simulink model "BugE_v0_40_MAS_loads_reg"  (R2015b)
settings: Solver=FixedStepDiscrete  StartTime=0.0  StopTime=1370  FixedStep=sample_time  RelTol=1e-3
values from neighbouring files (symbols this model uses):
  AB_diode_dV = 0.9    [main_sync.m]
  air_density = 1.225    [main_sync.m]
  bus_ac_Pmax_abs = 240    [main_sync.m]
  bus_charger_Pmax = 1000    [main_sync.m]
  bus_load_Pmax_abs = 260    [main_sync.m]
  capInitVolt = capVmax*sqrt(capInitSoC)    [main_sync.m]
  cyc_kph = [cyc_kph(:,1), cyc_kph(:,2)*speed_max_limit/speed_max]    [main_sync.m]
  cyc_repeat = 0    [main_sync.m]
  ess1_init_soc = 1    [main_sync.m]
  ess1_soh = 1    [main_sync.m]
  ess2_init_soc = 1    [main_sync.m]
  ess2_soh = 1    [main_sync.m]
  ess3_init_soc = 1    [main_sync.m]
  ess3_soh = 1    [main_sync.m]
  ess4_init_soc = 1    [main_sync.m]
  ess4_soh = 1    [main_sync.m]
  ess5_init_soc = 1    [main_sync.m]
  ess5_soh = 1    [main_sync.m]
  gear_ratio = 6    [main_sync.m]
  JADE_on = 0    [main_sync.m]
  loadpower = rawcsv(:,2)    [main_sync.m]
  loadtime = rawcsv(:,1)    [main_sync.m]
  lockSOCs = 0    [main_sync.m]
  max_brk_torque = 300    [main_sync.m]
  no_wheels = 3    [main_sync.m]
  period2 = max(loadtime)    [main_sync.m]
  PV_Pmax = 100    [main_sync.m]
  sample_time = 0.01    [main_sync.m]
  startup_seq_step_delay = 0.2    [main_sync.m]
  stop_option = 0    [main_sync.m]
  use_drive_cycle = 1    [main_sync.m]
  use_real_subs_loads = 1    [main_sync.m]
  vbus_max = 25    [main_sync.m]
  vbus_min = 17    [main_sync.m]
  vbus_safety_threshold = 2    [main_sync.m]
  vbus_threshold = 20    [main_sync.m]
  veh_CD = 0.35    [main_sync.m]
  veh_FA = 1.543    [main_sync.m]
  veh_gravity = 9.81*veh_mass    (= 1863.9)    [main_sync.m]
  veh_mass = 190    [main_sync.m]
  wh_1st_rrc = 0.02    [main_sync.m]
  wh_bearing_frc = 0.0015    [main_sync.m]
  wh_inertia = 0.0556    [main_sync.m]
  wh_radius = 0.508/2    (= 0.254)    [main_sync.m]
undefined symbols (not defined in the file or in its folder): capC, capR, cyc_acc, cyc_avg_time_samples, cyc_brk, cyc_grade, cyc_key, DCM_eff_factor_for_Vin, DCM_eff_for_Iout, DCM_Iout, DCM_Iout_max, DCM_Pin_noload, DCM_Pout_max, DCM_Vin, DCM_Vout, DiscIntNeverNeededParam, ess2_coulombic_eff, ess2_Ineg_max_SOC, ess2_Ineg_max_temp, ess2_Ipos_max_SOC, ess2_Ipos_max_temp, ess2_max_ah_cap, ess2_max_volts, ess2_min_volts, ess2_module_parallel, ess2_module_series, ess2_r_dis, ess2_soc, ess2_SOC_for_Ilimit, ess2_temp_for_Ilimit, ess2_temp_max, ess2_tmp, ess2_voc, ess3_coulombic_eff, ess3_max_ah_cap, ess3_module_parallel, ess3_module_series, ess3_r_dis, ess3_soc, ess3_tmp, ess3_voc, ess_coulombic_eff, ess_Ineg_max_SOC, ess_Ineg_max_temp, ess_Ipos_max_SOC, ess_Ipos_max_temp, ess_max_ah_cap, ess_max_volts, ess_min_volts, ess_module_parallel, ess_module_series, ess_nominal_volts, ess_r_dis, ess_soc, ess_SOC_for_Ilimit, ess_temp_for_Ilimit, ess_temp_max, ess_tmp, ess_voc, MC_eff1 ... (+18)
libraries: simulink x140, commfilt2 x1, simulink_extras x1
(part 3 of 7)

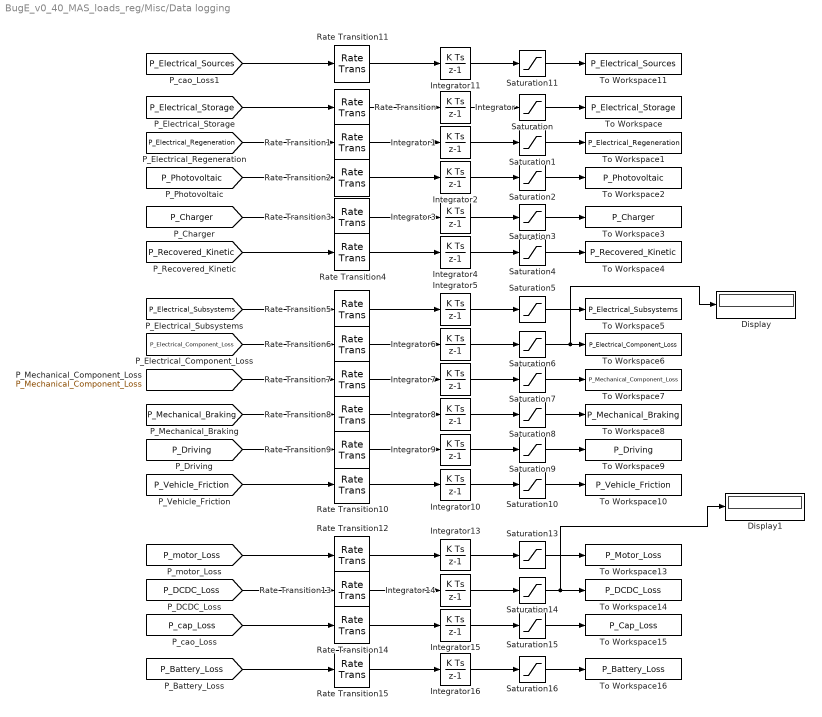
== system BugE_v0_40_MAS_loads_reg/Misc/Data logging ==
  Display : Display
  Display1 : Display
  Integrator{,1..11,13..16} (16 alike) : DiscreteIntegrator  InitialConditionSetting=State (most efficient)  ICPrevOutput=DiscIntNeverNeededParam  ICPrevScaledInput=DiscIntNeverNeededParam
  Rate Transition{,1..15} (16 alike) : RateTransition
  Saturation{,1..11,13..16} (16 alike) : Saturate  UpperLimit=inf  LowerLimit=0
  To Workspace : ToWorkspace  VariableName=P_Electrical_Storage  SampleTime=-1
      settings: MaxDataPoints=1
  To Workspace1 : ToWorkspace  VariableName=P_Electrical_Regeneration  SampleTime=-1
      settings: MaxDataPoints=1
  To Workspace10 : ToWorkspace  VariableName=P_Vehicle_Friction  SampleTime=-1
      settings: MaxDataPoints=1
  To Workspace11 : ToWorkspace  VariableName=P_Electrical_Sources  SampleTime=-1
      settings: MaxDataPoints=1
  To Workspace13 : ToWorkspace  VariableName=P_Motor_Loss  SampleTime=-1
      settings: MaxDataPoints=1
  To Workspace14 : ToWorkspace  VariableName=P_DCDC_Loss  SampleTime=-1
      settings: MaxDataPoints=1
  To Workspace15 : ToWorkspace  VariableName=P_Cap_Loss  SampleTime=-1
      settings: MaxDataPoints=1
  To Workspace16 : ToWorkspace  VariableName=P_Battery_Loss  SampleTime=-1
      settings: MaxDataPoints=1
  To Workspace2 : ToWorkspace  VariableName=P_Photovoltaic  SampleTime=-1
      settings: MaxDataPoints=1
  To Workspace3 : ToWorkspace  VariableName=P_Charger  SampleTime=-1
      settings: MaxDataPoints=1
  To Workspace4 : ToWorkspace  VariableName=P_Recovered_Kinetic  SampleTime=-1
      settings: MaxDataPoints=1
  To Workspace5 : ToWorkspace  VariableName=P_Electrical_Subsystems  SampleTime=-1
      settings: MaxDataPoints=1
  To Workspace6 : ToWorkspace  VariableName=P_Electrical_Component_Loss  SampleTime=-1
      settings: MaxDataPoints=1
  To Workspace7 : ToWorkspace  VariableName=P_Mechanical_Component_Loss  SampleTime=-1
      settings: MaxDataPoints=1
  To Workspace8 : ToWorkspace  VariableName=P_Mechanical_Braking  SampleTime=-1
      settings: MaxDataPoints=1
  To Workspace9 : ToWorkspace  VariableName=P_Driving  SampleTime=-1
      settings: MaxDataPoints=1
  wires:
  [P_Electrical_Storage] -> Rate Transition/1
  [P_Electrical_Regeneration] -> Rate Transition1/1
  [P_Photovoltaic] -> Rate Transition2/1
  [P_Charger] -> Rate Transition3/1
  [P_Recovered_Kinetic] -> Rate Transition4/1
  [P_Electrical_Subsystems] -> Rate Transition5/1
  [P_Electrical_Component_Loss] -> Rate Transition6/1
  [P_Mechanical_Component_Loss] -> Rate Transition7/1
  [P_Mechanical_Braking] -> Rate Transition8/1
  [P_Driving] -> Rate Transition9/1
  [P_Vehicle_Friction] -> Rate Transition10/1
  Integrator/1 -> Saturation/1
  Integrator1/1 -> Saturation1/1
  Integrator2/1 -> Saturation2/1
  Integrator3/1 -> Saturation3/1
  Integrator4/1 -> Saturation4/1
  Integrator5/1 -> Saturation5/1
  Integrator6/1 -> Saturation6/1
  Integrator7/1 -> Saturation7/1
  Integrator8/1 -> Saturation8/1
  Integrator9/1 -> Saturation9/1
  Integrator10/1 -> Saturation10/1
  Saturation/1 -> To Workspace/1
  Saturation1/1 -> To Workspace1/1
  Saturation2/1 -> To Workspace2/1
  Saturation3/1 -> To Workspace3/1
  Saturation4/1 -> To Workspace4/1
  Saturation5/1 -> To Workspace5/1
  Saturation6/1 -> Display/1, To Workspace6/1
  Saturation7/1 -> To Workspace7/1
  Saturation8/1 -> To Workspace8/1
  Saturation9/1 -> To Workspace9/1
  Saturation10/1 -> To Workspace10/1
  Rate Transition/1 -> Integrator/1
  Rate Transition1/1 -> Integrator1/1
  Rate Transition2/1 -> Integrator2/1
  Rate Transition3/1 -> Integrator3/1
  Rate Transition4/1 -> Integrator4/1
  Rate Transition5/1 -> Integrator5/1
  Rate Transition6/1 -> Integrator6/1
  Rate Transition7/1 -> Integrator7/1
  Rate Transition8/1 -> Integrator8/1
  Rate Transition9/1 -> Integrator9/1
  Rate Transition10/1 -> Integrator10/1
  [P_DCDC_Loss] -> Rate Transition13/1
  [P_cap_Loss] -> Rate Transition14/1
  [P_Battery_Loss] -> Rate Transition15/1
  Integrator14/1 -> Saturation14/1
  Integrator15/1 -> Saturation15/1
  Integrator16/1 -> Saturation16/1
  Saturation14/1 -> Display1/1, To Workspace14/1
  Saturation15/1 -> To Workspace15/1
  Saturation16/1 -> To Workspace16/1
  Rate Transition13/1 -> Integrator14/1
  Rate Transition14/1 -> Integrator15/1
  Rate Transition15/1 -> Integrator16/1
  Saturation13/1 -> To Workspace13/1
  Integrator13/1 -> Saturation13/1
  Rate Transition12/1 -> Integrator13/1
  [P_motor_Loss] -> Rate Transition12/1
  Saturation11/1 -> To Workspace11/1
  Integrator11/1 -> Saturation11/1
  Rate Transition11/1 -> Integrator11/1
  [P_Electrical_Sources] -> Rate Transition11/1

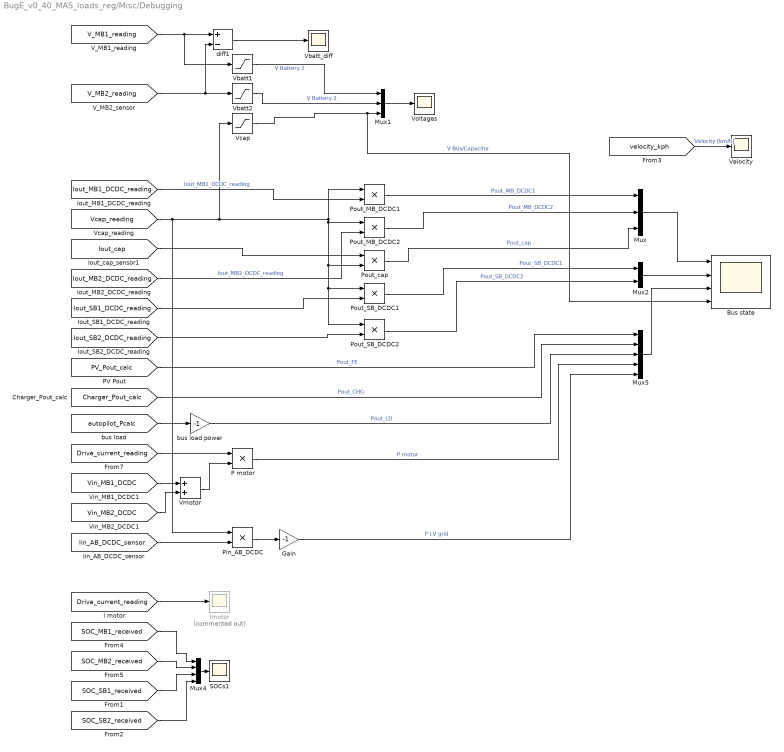
== system BugE_v0_40_MAS_loads_reg/Misc/Debugging ==
  Bus state : Scope  NumInputPorts=4
  Gain : Gain  Gain=-1
  Imotor : Scope  Commented=on
  Mux : Mux  Inputs=3
  Mux1 : Mux  Inputs=3
  Mux2 : Mux  Inputs=2
  Mux4 : Mux
  Mux5 : Mux  Inputs=5
  P motor : Product
  Pin_AB_DCDC : Product
  Pout_MB_DCDC1 : Product
  Pout_MB_DCDC2 : Product
  Pout_SB_DCDC1 : Product
  Pout_SB_DCDC2 : Product
  Pout_cap : Product
  SOCs1 : Scope
  Vbatt1 : Saturate  UpperLimit=100  LowerLimit=-100
  Vbatt2 : Saturate  UpperLimit=100  LowerLimit=-100
  Vbatt_diff : Scope
  Vcap : Saturate  UpperLimit=100  LowerLimit=-100
  Velocity : Scope
  Vmotor : Sum
  Voltages : Scope
  bus load power : Gain  Gain=-1
  diff1 : Sum  Inputs=+-
  wires:
  [V_MB2_reading] -> diff1/2, Vbatt2/1
  [Vcap_reading] -> Pout_SB_DCDC2/1, Pout_SB_DCDC1/1, Pout_cap/2, Pout_MB_DCDC2/1, Pout_MB_DCDC1/1, Vcap/1, Pin_AB_DCDC/1
  [Iout_cap] -> Pout_cap/1
  Vbatt1/1 -> Mux1/1  "V Battery 1"
  Vbatt2/1 -> Mux1/2  "V Battery 2"
  Vcap/1 -> Bus state/4, Mux1/3  "V Bus/Capacitor"
  [Iout_MB2_DCDC_reading] -> Pout_MB_DCDC2/2  "Iout_MB2_DCDC_reading"
  diff1/1 -> Vbatt_diff/1
  Mux1/1 -> Voltages/1
  [velocity_kph] -> Velocity/1  "Velocity [km/h]"
  [V_MB1_reading] -> Vbatt1/1, diff1/1
  [Iout_MB1_DCDC_reading] -> Pout_MB_DCDC1/2  "Iout_MB1_DCDC_reading"
  Pout_cap/1 -> Mux/3  "Pout_cap"
  Mux4/1 -> SOCs1/1
  [SOC_MB2_received] -> Mux4/2
  [SOC_MB1_received] -> Mux4/1
  [Drive_current_reading] -> Imotor/1
  [Iout_SB1_DCDC_reading] -> Pout_SB_DCDC1/2
  [Iout_SB2_DCDC_reading] -> Pout_SB_DCDC2/2
  [PV_Pout_calc] -> Mux5/1  "Pout_FE"
  Pout_MB_DCDC1/1 -> Mux/1  "Pout_MB_DCDC1"
  Pout_SB_DCDC1/1 -> Mux2/1  "Pout_SB_DCDC1"
  Pout_SB_DCDC2/1 -> Mux2/2  "Pout_SB_DCDC2"
  Pout_MB_DCDC2/1 -> Mux/2  "Pout_MB_DCDC2"
  [Charger_Pout_calc] -> Mux5/2  "Pout_CHG"
  Mux/1 -> Bus state/1
  [autopilot_Pcalc] -> bus load power/1
  bus load power/1 -> Mux5/3  "Pout_LD"
  Mux2/1 -> Bus state/2
  Mux5/1 -> Bus state/3
  [Vin_MB1_DCDC] -> Vmotor/1
  [Vin_MB2_DCDC] -> Vmotor/2
  [Drive_current_reading] -> P motor/1
  Vmotor/1 -> P motor/2
  P motor/1 -> Mux5/4  "P motor"
  [Iin_AB_DCDC_sensor] -> Pin_AB_DCDC/2
  Pin_AB_DCDC/1 -> Gain/1
  Gain/1 -> Mux5/5  "P LV grid"
  [SOC_SB1_received] -> Mux4/3
  [SOC_SB2_received] -> Mux4/4

== system BugE_v0_40_MAS_loads_reg/Misc/Energy Calculations ==
  Battery losses : Subsystem
  Battery regen : Subsystem
  DCDC losses : Subsystem
  E_accessories : Subsystem
  E_battery_total : Subsystem
  E_cap_total : Subsystem
  E_vehicle_drive : Subsystem
  E_vehicle_friction : Subsystem
  Powertrain mech. losses : Subsystem
  electrical components : Sum  Inputs=++++
  electrical sinks : Sum  Inputs=8
  electrical sources : Sum  Inputs=5
  electrical subsystems : Sum
  mechanical sinks : Sum  Inputs=4
  mechanical sources : Sum  Inputs=-++
  net electrical storage : Sum  Inputs=++--
  tag scope: P_Battery_Loss=global, P_Charger=global, P_DCDC_Loss=global, P_Driving=global, P_Electrical_Component_Loss=global, P_Electrical_Regeneration=global, P_Electrical_Sources=global, P_Electrical_Storage=global, P_Electrical_Subsystems=global, P_Mechanical_Braking=global, P_Mechanical_Component_Loss=global, P_Photovoltaic=global, P_Recovered_Kinetic=global, P_Vehicle_Friction=global, P_cap_Loss=global, P_motor_Loss=global
  wires:
  Powertrain mech. losses/1(Out1) -> [P_Mechanical_Component_Loss], mechanical sinks/1
  [E_mech_brake] -> mechanical sinks/2, [P_Mechanical_Braking]
  electrical sinks/1 -> mechanical sources/2
  mechanical sinks/1 -> mechanical sources/3
  E_vehicle_drive/1(Out1) -> [P_Driving], mechanical sinks/3
  E_vehicle_friction/1(Out1) -> [P_Vehicle_Friction], mechanical sinks/4
  [E_cap_loss] -> [P_cap_Loss], electrical components/4, electrical sinks/8
  [E_cap_regen] -> electrical sinks/1, net electrical storage/3
  Battery regen/1(Out1) -> net electrical storage/4, electrical sinks/2
  Battery losses/1(Out1) -> [P_Battery_Loss], electrical components/3, electrical sinks/7
  [E_motor_eff] -> electrical sinks/5, [P_motor_Loss], electrical components/1
  [E_autopilot] -> electrical subsystems/2, electrical sinks/4
  [E_charger] -> [P_Charger], electrical sources/5
  [E_PV] -> [P_Photovoltaic], electrical sources/4
  E_cap_total/1(Out1) -> net electrical storage/1, electrical sources/1
  E_battery_total/1(Out1) -> net electrical storage/2, electrical sources/2
  [E_motor_regen] -> [P_Electrical_Regeneration], electrical sources/3
  DCDC losses/1(Out1) -> [P_DCDC_Loss], electrical components/2, electrical sinks/6
  E_accessories/1(Out1) -> electrical sinks/3, electrical subsystems/1
  mechanical sources/1 -> [P_Recovered_Kinetic]
  net electrical storage/1 -> [P_Electrical_Storage]
  electrical subsystems/1 -> [P_Electrical_Subsystems]
  electrical components/1 -> [P_Electrical_Component_Loss]
  electrical sources/1 -> [P_Electrical_Sources], mechanical sources/1

== system BugE_v0_40_MAS_loads_reg/Misc/STOP Sim ==
  note: stop on: 0 SOC, 1 both, 2 Vbatt, 3 nothing
  note: STOP SIMULATION / SEND STOP-BATTERY SIGNALS
  Logical Operator : Logic  AllPortsSameDT=off  OutDataTypeStr=boolean
  Logical Operator1 : Logic  Operator=OR  AllPortsSameDT=off  OutDataTypeStr=boolean
  Stop Simulation : Stop
  Switch2 : MultiPortSwitch  DataPortOrder=Zero-based contiguous  Inputs=4
  Switch3 : MultiPortSwitch  DataPortOrder=Zero-based contiguous  Inputs=4
  don't stop : Constant  Value=0
  ess min V : Constant  Value=ess_min_volts*ess_module_series
  min SOC : Constant  Value=0.001
  or1 : Logic  Operator=OR  AllPortsSameDT=off  OutDataTypeStr=boolean
  or2 : Logic  Operator=OR  AllPortsSameDT=off  OutDataTypeStr=boolean
  stopB1_SOC : RelationalOperator  Operator=<=  OutDataTypeStr=boolean
  stopB1_Vmin : RelationalOperator  Operator=<=  OutDataTypeStr=boolean
  stopB2_SOC : RelationalOperator  Operator=<=  OutDataTypeStr=boolean
  stopB2_Vmin : RelationalOperator  Operator=<=  OutDataTypeStr=boolean
  stop_option : Constant  Value=stop_option
  wires:
  min SOC/1 -> stopB2_SOC/1, stopB1_SOC/2
  [SOC_MB1] -> stopB1_SOC/1
  [SOC_MB2] -> stopB2_SOC/2
  [V_MB1_reading] -> stopB1_Vmin/1
  ess min V/1 -> stopB1_Vmin/2, stopB2_Vmin/1
  [V_MB2_reading] -> stopB2_Vmin/2
  stopB1_SOC/1 -> Switch2/2, or1/1
  stopB1_Vmin/1 -> or1/2, Switch2/4
  stopB2_SOC/1 -> Switch3/2, or2/1
  stopB2_Vmin/1 -> or2/2, Switch3/4
  Switch2/1 -> Logical Operator/1
  Switch3/1 -> Logical Operator/2
  Logical Operator1/1 -> Stop Simulation/1
  or1/1 -> Switch2/3
  or2/1 -> Switch3/3
  stop_option/1 -> Switch3/1, Switch2/1
  don't stop/1 -> Switch2/5, Switch3/5
  Logical Operator/1 -> Logical Operator1/1
  [endcycle_stopsim] -> Logical Operator1/2

== system BugE_v0_40_MAS_loads_reg/Motor-Generator Drive (HV Grid)/Current limiter ==
  note: Enforce physical limits of
      | DCDCs in MB failure mode
  Input power [W] : Inport
  Voltage [V] : Inport  Port=2
  Req. torque : Inport  Port=3
  Abs : Abs
  Compare : simulink/Logic and Bit Operations/Compare To Constant  relop===  const=1  OutDataTypeStr=boolean
  DAB_Imax : Constant  Value=MC_Imax  SampleTime=sample_time
  Goto : Goto  Commented=on  GotoTag=Pmax_motor  TagVisibility=global
  I max motor : Constant  Value=mc_max_crrnt  SampleTime=sample_time
  Max : MinMax  Function=max
  MinMax: I <= I_max : MinMax  Inputs=2
  Multiply1 : Product  Inputs=**
  Multiply2 : Product  Inputs=**
  Multiply3 : Product  Inputs=*/*
  Scope : Scope
  Sign : Signum
  Unit Delay prevent timing errors : UnitDelay  SampleTime=sample_time
  failure mode selector : Switch  Criteria=u2 > Threshold
  todouble : DataTypeConversion  OutDataTypeStr=double
  Limited input power : Outport
  Limited torque : Outport  Port=2
  wires:
  Abs/1 -> MinMax: I <= I_max/2
  Voltage [V]/1 -> Multiply1/2
  Multiply1/1 -> Goto/1, MinMax: I <= I_max/1
  Multiply2/1 -> Multiply3/1, Limited input power/1
  Input power [W]/1 -> Multiply3/2, Sign/1, Abs/1
  Sign/1 -> Scope/1, Multiply2/2
  MinMax: I <= I_max/1 -> Multiply2/1
  Req. torque/1 -> Multiply3/3
  Multiply3/1 -> Limited torque/1
  [MB_DCDC_command_type] -> Unit Delay prevent timing errors/1
  Max/1 -> Compare/1
  Compare/1 -> failure mode selector/2
  I max motor/1 -> failure mode selector/3
  failure mode selector/1 -> Multiply1/1
  todouble/1 -> Max/1
  Unit Delay prevent timing errors/1 -> todouble/1
  DAB_Imax/1 -> failure mode selector/1

== system BugE_v0_40_MAS_loads_reg/Motor-Generator Drive (HV Grid)/Energy Quantification ==
  Pin : Inport
  speed : Inport  Port=2
  torque out : Inport  Port=3
  inertia torque : Inport  Port=4
  < 0 : Saturate  UpperLimit=0  LowerLimit=-inf
  > 0 : Saturate  UpperLimit=inf  LowerLimit=0
  Abs : Abs
  Gain : Gain  Gain=-1
  Inertia power : Product  SaturateOnIntegerOverflow=on  RndMeth=Zero  InputSameDT=on  OutDataTypeStr=Inherit: Same as first input
  Lost power : Sum  Inputs=+--
  Mech power : Product  Inputs=**  SaturateOnIntegerOverflow=on  RndMeth=Zero  InputSameDT=on  OutDataTypeStr=Inherit: Same as first input
  Switch : Switch  Criteria=u2 > Threshold
  add : Sum  Inputs=2
  tag scope: E_motor_eff=global, E_motor_inertia=global, E_motor_regen=global
  wires:
  speed/1 -> Mech power/1, Inertia power/1
  > 0/1 -> [E_motor_inertia]
  torque out/1 -> Mech power/2
  Inertia power/1 -> > 0/1, Lost power/3
  Abs/1 -> [E_motor_eff], add/2
  Lost power/1 -> Abs/1
  Mech power/1 -> Lost power/2
  Pin/1 -> Lost power/1, < 0/1
  inertia torque/1 -> Inertia power/2
  Gain/1 -> add/1, Switch/3, Switch/2
  < 0/1 -> Gain/1
  add/1 -> Switch/1
  Switch/1 -> [E_motor_regen]

== system BugE_v0_40_MAS_loads_reg/Motor-Generator Drive (HV Grid)/Torque limiter ==
  Speed [rad/s] : Inport
  Inertia torque [Nm] : Inport  Port=2
  Requested throttle [0-1] : Inport  Port=3
  >=0 : simulink/Logic and Bit Operations/Compare To Zero  relop=>=  OutDataTypeStr=boolean
  Available torque : Sum  Inputs=+-
  Max generator torque : Lookup_n-D  NumberOfTableDimensions=1  BreakpointsForDimension1=mc_map_spd*mc_spd_scale  Table=mc_max_gen_trq*mc_trq_scale  DiagnosticForOutOfRangeInput=Warning  InternalRulePriority=Speed  SaturateOnIntegerOverflow=on  InputSameDT=on
  Max motor torque : Lookup_n-D  NumberOfTableDimensions=1  BreakpointsForDimension1=mc_map_spd*mc_spd_scale  Table=mc_max_trq*mc_trq_scale  InternalRulePriority=Speed  SaturateOnIntegerOverflow=on  InputSameDT=on
  MinMax : MinMax  Inputs=2
  MinMax1 : MinMax  Function=max  Inputs=2
  "Motor_torque_req " : Switch  Criteria=u2 > Threshold
  Product : Product
  Requested torque : Sum
  Switch: limit torque : Switch  Criteria=u2 > Threshold
  Limited req. trq : Outport
  wires:
  Max motor torque/1 -> Available torque/1, MinMax/2
  Available torque/1 -> Product/1
  Inertia torque [Nm]/1 -> Requested torque/1, Available torque/2
  Requested torque/1 -> MinMax1/2, >=0/1, MinMax/1
  Requested throttle [0-1]/1 -> Product/2
  Max generator torque/1 -> MinMax1/1
  >=0/1 -> Switch: limit torque/2
  MinMax/1 -> Switch: limit torque/1
  MinMax1/1 -> Switch: limit torque/3
  Switch: limit torque/1 -> Limited req. trq/1
  Speed [rad/s]/1 -> Max generator torque/1, Max motor torque/1
  Product/1 -> "Motor_torque_req "/2, "Motor_torque_req "/1
  "Motor_torque_req "/1 -> Requested torque/2
  [Generator_torque] -> "Motor_torque_req "/3

== system BugE_v0_40_MAS_loads_reg/Vehicle/Achievable vehicle speed ==
  Vehicle speed at the beginning of the time step [m/s] : Inport
  Available avg. tractive force [N] : Inport  Port=2
  2a : Gain  Gain=2
  4ac : Gain  Gain=4
  Add2 : Sum
  Climbing force : Product  Inputs=3
  Energy Quantification1 : Subsystem
  Gain : Gain  Gain=1/2
  Half the aerodynamic drag at the beginning of the time step : Product
  Product1 : Product
  Saturation : Saturate  UpperLimit=1000  LowerLimit=0
  Tire roll drag force : Product  Inputs=****
  Trig Fn : Trigonometry  Operator=cos
  Trig Fn2 : Trigonometry
  ac : Product  Inputs=**  SaturateOnIntegerOverflow=on  RndMeth=Zero  InputSameDT=on  OutDataTypeStr=Inherit: Same as first input
  aero1 : Constant  Value=0.5*air_density*veh_CD*veh_FA  SampleTime=sample_time
  aero2 : Constant  Value=0.5*air_density*veh_CD*veh_FA  SampleTime=sample_time
  angle of elevation : Trigonometry  Operator=atan
  b^2 : Product  Inputs=**  SaturateOnIntegerOverflow=on  RndMeth=Zero  InputSameDT=on  OutDataTypeStr=Inherit: Same as first input
  delta : Sum  Inputs=+-
  m*v_prev/dt : Product  Inputs=**  SaturateOnIntegerOverflow=on  RndMeth=Zero  InputSameDT=on  OutDataTypeStr=Inherit: Same as first input
  quadratic_a : Gain  Gain=1/2
  quadratic_b : Product  Inputs=*/  SaturateOnIntegerOverflow=on  RndMeth=Zero  InputSameDT=on  OutDataTypeStr=Inherit: Same as first input
  quadratic_c : Sum  Inputs=-++-
  sol : Product  Inputs=/*
  sqrt(delta) : Sqrt  SaturateOnIntegerOverflow=on
  sqrt(delta)-b : Sum  Inputs=-+
  todouble : DataTypeConversion  OutDataTypeStr=double
  u>0 : Fcn  Expr=u>0
  veh_gravity : Constant  Value=veh_gravity  SampleTime=sample_time
  veh_mass : Constant  Value=veh_mass  SampleTime=sample_time
  wh_1st_rrc : Constant  Value=wh_1st_rrc  SampleTime=sample_time
  Vehicle speed at the end of time step [m/s] : Outport
  wires:
  Half the aerodynamic drag at the beginning of the time step/1 -> quadratic_c/2
  Product1/1 -> Gain/1
  aero2/1 -> quadratic_a/1
  Gain/1 -> Half the aerodynamic drag at the beginning of the time step/2
  Add2/1 -> quadratic_c/3
  veh_gravity/1 -> Climbing force/3, Tire roll drag force/4
  Trig Fn/1 -> Tire roll drag force/3
  wh_1st_rrc/1 -> Tire roll drag force/2
  u>0/1 -> Tire roll drag force/1, Climbing force/1
  angle of elevation/1 -> Trig Fn2/1, Trig Fn/1
  m*v_prev/dt/1 -> quadratic_c/1
  [grade] -> angle of elevation/1
  veh_mass/1 -> quadratic_b/1
  aero1/1 -> Half the aerodynamic drag at the beginning of the time step/1
  Trig Fn2/1 -> Climbing force/2
  [dt] -> todouble/1
  Available avg. tractive force [N]/1 -> quadratic_c/4, Energy Quantification1/3(Ftract)
  Tire roll drag force/1 -> Energy Quantification1/1(Froll), Add2/1
  Climbing force/1 -> Energy Quantification1/2(Fclimb), Add2/2
  Vehicle speed at the beginning of the time step [m/s]/1 -> Energy Quantification1/4(Vi), u>0/1, Product1/2, m*v_prev/dt/2, Product1/1
  Saturation/1 -> Vehicle speed at the end of time step [m/s]/1
  quadratic_c/1 -> ac/2
  quadratic_b/1 -> b^2/2, sqrt(delta)-b/1, b^2/1, m*v_prev/dt/1
  ac/1 -> 4ac/1
  4ac/1 -> delta/2
  b^2/1 -> delta/1
  delta/1 -> sqrt(delta)/1
  sqrt(delta)/1 -> sqrt(delta)-b/2
  sqrt(delta)-b/1 -> sol/2
  2a/1 -> sol/1
  quadratic_a/1 -> 2a/1, ac/1
  sol/1 -> Saturation/1
  todouble/1 -> quadratic_b/2

== system BugE_v0_40_MAS_loads_reg/Auxiliaries (LV Grid)/AB (w// diode)/Calculate SOC ==
  Temp [C] : Inport
  I [A] : Inport  Port=2
  1/3600 : Gain  Gain=1/3600
  Add : Sum  Inputs=-+
  Constant1 : Constant  SampleTime=sample_time
  Coulombic efficiency : Lookup_n-D  NumberOfTableDimensions=1  BreakpointsForDimension1=ess3_tmp  Table=ess3_coulombic_eff  InternalRulePriority=Speed  SaturateOnIntegerOverflow=on  InputSameDT=on
  Energy left [Ah] : Sum  Inputs=-+
  I adjusted : Product
  Max capacity [Ah] w/ SOH : Lookup_n-D  NumberOfTableDimensions=1  BreakpointsForDimension1=ess3_tmp  Table=ess3_max_ah_cap*ess5_soh  InternalRulePriority=Speed  SaturateOnIntegerOverflow=on  InputSameDT=on
  Multiply : Product
  Multiply1 : Product
  Resettable Integrator : Subsystem
  "SOC " : Product  Inputs=*/
  Saturation : Saturate  UpperLimit=1  LowerLimit=0
  Switch : Switch  Criteria=u2 > Threshold
  ess2_modules : Constant  Value=ess2_module_series*ess2_module_parallel  SampleTime=sample_time
  SOC : Outport
  wires:
  Resettable Integrator/1(Out1) -> Energy left [Ah]/1
  I [A]/1 -> Switch/2, Switch/1, I adjusted/1
  Switch/1 -> 1/3600/1
  Coulombic efficiency/1 -> I adjusted/2
  Energy left [Ah]/1 -> "SOC "/1
  I adjusted/1 -> Switch/3
  1/3600/1 -> Resettable Integrator/1(input)
  Temp [C]/1 -> Max capacity [Ah] w/ SOH/1, Coulombic efficiency/1
  Multiply1/1 -> Multiply/2, "SOC "/2, Energy left [Ah]/2
  "SOC "/1 -> Saturation/1
  Constant1/1 -> Add/2
  Multiply/1 -> Resettable Integrator/2(IC)
  Add/1 -> Multiply/1
  Saturation/1 -> SOC/1
  ess2_modules/1 -> Multiply1/2
  Max capacity [Ah] w/ SOH/1 -> Multiply1/1
  [AB_SOCinit] -> Add/1

== system BugE_v0_40_MAS_loads_reg/Auxiliaries (LV Grid)/AB (w// diode)/Compute current (nolimit) ==
  Voc [V] : Inport
  Rint [Ohm] : Inport  Port=2
  Output power [W] : Inport  Port=3
  diode_dV [V] : Inport  Port=4
  -b-sqrt(D) : Sum  Inputs=+-
  2*a : Gain  Gain=2
  4*a*c : Gain  Gain=4
  I : Product  Inputs=*/
  I*R : Product  Inputs=**
  Subtract : Sum  Inputs=+-
  Terminator : Terminator
  V_AB : Sum  Inputs=+-
  Voc-Vdiode : Sum  Inputs=+-
  b^2 : Product
  b^2-4*a*c : Sum  Inputs=+-
  c*a : Product
  sqrt(Delta) : Sqrt  SaturateOnIntegerOverflow=on
  I [A] : Outport
  V_out [V] : Outport  Port=2
  wires:
  Output power [W]/1 -> c*a/1
  Voc-Vdiode/1 -> Subtract/1, -b-sqrt(D)/1, b^2/2, b^2/1
  Rint [Ohm]/1 -> c*a/2, 2*a/1, I*R/2
  c*a/1 -> 4*a*c/1
  b^2/1 -> b^2-4*a*c/1
  4*a*c/1 -> b^2-4*a*c/2
  b^2-4*a*c/1 -> sqrt(Delta)/1
  sqrt(Delta)/1 -> -b-sqrt(D)/2
  -b-sqrt(D)/1 -> I/1
  2*a/1 -> I/2
  I/1 -> I [A]/1, I*R/1
  I*R/1 -> Subtract/2, V_AB/2
  Subtract/1 -> V_out [V]/1
  diode_dV [V]/1 -> Voc-Vdiode/2
  Voc [V]/1 -> Voc-Vdiode/1, V_AB/1
  V_AB/1 -> Terminator/1

== system BugE_v0_40_MAS_loads_reg/Auxiliaries (LV Grid)/AB (w// diode)/Energy Quantification ==
  Vout : Inport
  Iout : Inport  Port=2
  R : Inport  Port=3
  diode_dV [V] : Inport  Port=4
  < 0 : Saturate  UpperLimit=0  LowerLimit=-inf
  > 0 : Saturate  UpperLimit=inf  LowerLimit=0  LinearizeAsGain=off
  Diode power : Product
  Gain : Gain  Gain=-1
  P_D+P_R : Sum
  Power : Product
  R power loss : Product  Inputs=3
  tag scope: E_batt_loss5=global, E_batt_regen5=global, E_batt_useful5=global
  wires:
  Vout/1 -> Power/1
  Iout/1 -> Power/2, Diode power/1, R power loss/2, R power loss/1
  Gain/1 -> [E_batt_regen5]
  Power/1 -> < 0/1, > 0/1
  < 0/1 -> Gain/1
  > 0/1 -> [E_batt_useful5]
  R power loss/1 -> P_D+P_R/1
  R/1 -> R power loss/3
  diode_dV [V]/1 -> Diode power/2
  Diode power/1 -> P_D+P_R/2
  P_D+P_R/1 -> [E_batt_loss5]

== system BugE_v0_40_MAS_loads_reg/Auxiliaries (LV Grid)/AB (w// diode)/Pack Voc, R ==
  Temp [degC] : Inport
  SOC_prev : Inport  Port=2
  Req. power [W] : Inport  Port=3
  >=0 : simulink/Logic and Bit Operations/Compare To Zero  relop=>=  OutDataTypeStr=boolean
  Product : Product  Inputs=3
  Product1 : Product  Inputs=/**/
  Product2 : Product  Inputs=/**/
  R_charge [Ohm] : Lookup_n-D  BreakpointsForDimension1=ess2_tmp  BreakpointsForDimension2=ess2_soc  Table=ess2_r_dis  InternalRulePriority=Speed  RndMeth=Simplest  InputSameDT=on
  R_discharge [Ohm] : Lookup_n-D  BreakpointsForDimension1=ess3_tmp  BreakpointsForDimension2=ess3_soc  Table=ess3_r_dis  InternalRulePriority=Speed  RndMeth=Simplest  InputSameDT=on
  Switch : Switch  Criteria=u2 > Threshold
  VOC [V] : Lookup_n-D  BreakpointsForDimension1=ess3_tmp  BreakpointsForDimension2=ess3_soc  Table=ess3_voc  InternalRulePriority=Speed  RndMeth=Simplest  InputSameDT=on
  ess3_module _parallel : Constant  Value=ess3_module_parallel  SampleTime=sample_time
  ess3_module _series : Constant  Value=ess3_module_series  SampleTime=sample_time
  ess5_soh : Constant  Value=ess5_soh  SampleTime=sample_time
  Pack Voc [V] : Outport
  Pack R [Ohm] : Outport  Port=2
  wires:
  Switch/1 -> Pack R [Ohm]/1
  Req. power [W]/1 -> >=0/1
  R_discharge [Ohm]/1 -> Product1/2
  Product/1 -> Pack Voc [V]/1
  VOC [V]/1 -> Product/2
  ess3_module _series/1 -> Product/3, Product2/2, Product1/3
  Temp [degC]/1 -> R_charge [Ohm]/1, R_discharge [Ohm]/1, VOC [V]/1
  SOC_prev/1 -> R_charge [Ohm]/2, R_discharge [Ohm]/2, VOC [V]/2
  ess5_soh/1 -> Product2/1, Product1/1, Product/1
  >=0/1 -> Switch/2
  ess3_module _parallel/1 -> Product1/4, Product2/4
  R_charge [Ohm]/1 -> Product2/3
  Product2/1 -> Switch/3
  Product1/1 -> Switch/1

== system BugE_v0_40_MAS_loads_reg/Auxiliaries (LV Grid)/AB DCDC/Energy Quantification ==
  In1 : Inport
  In2 : Inport  Port=2
  Abs1 : Abs
  Ploss DCM : Sum  Inputs=-+
  tag scope: E_DCM_loss=global
  wires:
  Abs1/1 -> [E_DCM_loss]
  Ploss DCM/1 -> Abs1/1
  In1/1 -> Ploss DCM/1
  In2/1 -> Ploss DCM/2

== system BugE_v0_40_MAS_loads_reg/Auxiliaries (LV Grid)/Auxiliary load (USB ports)/Energy Quantification ==
  Power : Inport
  tag scope: E_usb=global
  wires:
  Power/1 -> [E_usb]

== system BugE_v0_40_MAS_loads_reg/Auxiliaries (LV Grid)/Auxiliary load (lights)/Energy Quantification ==
  Power : Inport
  tag scope: E_accessories=global
  wires:
  Power/1 -> [E_accessories]

== system BugE_v0_40_MAS_loads_reg/Auxiliaries (LV Grid)/ECU & sensors load/Energy Quantification ==
  Power : Inport
  tag scope: E_ECU=global
  wires:
  Power/1 -> [E_ECU]

== system BugE_v0_40_MAS_loads_reg/Energy Storage (New Grid)/AC/Energy Quantification ==
  Power : Inport
  tag scope: E_ac=global
  wires:
  Power/1 -> [E_ac]

== system BugE_v0_40_MAS_loads_reg/Energy Storage (New Grid)/AutoPilot/Energy Quantification ==
  Power : Inport
  tag scope: E_autopilot=global
  wires:
  Power/1 -> [E_autopilot]

== system BugE_v0_40_MAS_loads_reg/Energy Storage (New Grid)/Capacitor/Energy Quantification ==
  R : Inport
  Vcap_RC : Inport  Port=2
  Iout : Inport  Port=3
  (I^2)R : Product  Inputs=***
  < 0 : Saturate  UpperLimit=0  LowerLimit=-inf  LinearizeAsGain=off
  > 0 : Saturate  UpperLimit=inf  LowerLimit=0  LinearizeAsGain=off
  Discrete-Time Integrator1 : DiscreteIntegrator  InitialConditionSetting=State (most efficient)  SampleTime=sample_time  ICPrevOutput=DiscIntNeverNeededParam  ICPrevScaledInput=DiscIntNeverNeededParam
  Discrete-Time Integrator2 : DiscreteIntegrator  InitialConditionSetting=State (most efficient)  SampleTime=sample_time  ICPrevOutput=DiscIntNeverNeededParam  ICPrevScaledInput=DiscIntNeverNeededParam
  Display1 : Display
  Display2 : Display
  Gain : Gain  Gain=-1
  Pout_RC1 : Product
  tag scope: E_cap_loss=global, E_cap_regen=global, E_cap_useful=global
  wires:
  Vcap_RC/1 -> Pout_RC1/2
  R/1 -> (I^2)R/1
  > 0/1 -> [E_cap_useful]
  Pout_RC1/1 -> Discrete-Time Integrator2/1, < 0/1, > 0/1
  Iout/1 -> Pout_RC1/1, (I^2)R/2, (I^2)R/3
  (I^2)R/1 -> Discrete-Time Integrator1/1, [E_cap_loss]
  Gain/1 -> [E_cap_regen]
  < 0/1 -> Gain/1
  Discrete-Time Integrator1/1 -> Display1/1  "E cap loss"
  Discrete-Time Integrator2/1 -> Display2/1  "E cap out"

== system BugE_v0_40_MAS_loads_reg/Energy Storage (New Grid)/Charger/Energy Quantification ==
  Power : Inport
  tag scope: E_charger=global
  wires:
  Power/1 -> [E_charger]

== system BugE_v0_40_MAS_loads_reg/Energy Storage (New Grid)/MB1/Calculate SOC ==
  Temp [C] : Inport
  I [A] : Inport  Port=2
  1/3600 : Gain  Gain=1/3600
  Add : Sum  Inputs=-+
  Constant1 : Constant  SampleTime=sample_time
  Coulombic efficiency : Lookup_n-D  NumberOfTableDimensions=1  BreakpointsForDimension1=ess_tmp  Table=ess_coulombic_eff  InternalRulePriority=Speed  SaturateOnIntegerOverflow=on  InputSameDT=on
  Energy left [Ah] : Sum  Inputs=-+
  I adjusted : Product
  Max capacity [Ah] w/ SOH : Lookup_n-D  NumberOfTableDimensions=1  BreakpointsForDimension1=ess_tmp  Table=ess_max_ah_cap*ess1_soh  InternalRulePriority=Speed  SaturateOnIntegerOverflow=on  InputSameDT=on
  Multiply : Product
  Multiply1 : Product
  Resettable Integrator : Subsystem
  "SOC " : Product  Inputs=*/
  Saturation : Saturate  UpperLimit=1  LowerLimit=0
  Switch : Switch  Criteria=u2 > Threshold
  Switch1 : Switch  Criteria=u2 > Threshold
  ess_modules : Constant  Value=ess_module_series*ess_module_parallel  SampleTime=sample_time
  lockSOCs : Constant  Value=lockSOCs
  SOC : Outport
  wires:
  Resettable Integrator/1(Out1) -> Energy left [Ah]/1
  I [A]/1 -> Switch/1, Switch/2, I adjusted/1
  Switch/1 -> 1/3600/1
  Coulombic efficiency/1 -> I adjusted/2
  Energy left [Ah]/1 -> "SOC "/1
  I adjusted/1 -> Switch/3
  1/3600/1 -> Resettable Integrator/1(input)
  Temp [C]/1 -> Max capacity [Ah] w/ SOH/1, Coulombic efficiency/1
  Multiply1/1 -> Multiply/2, "SOC "/2, Energy left [Ah]/2
  "SOC "/1 -> Saturation/1
  [MB1_SOCinit] -> Add/1, Switch1/1
  Constant1/1 -> Add/2
  Multiply/1 -> Resettable Integrator/2(IC)
  Add/1 -> Multiply/1
  Saturation/1 -> Switch1/3
  ess_modules/1 -> Multiply1/2
  Max capacity [Ah] w/ SOH/1 -> Multiply1/1
  lockSOCs/1 -> Switch1/2
  Switch1/1 -> SOC/1

== system BugE_v0_40_MAS_loads_reg/Energy Storage (New Grid)/MB1/Compute current (nolimit) ==
  Voc [V] : Inport
  Rint [Ohm] : Inport  Port=2
  Output power [W] : Inport  Port=3
  2*R : Gain  Gain=2
  4*R*Pbty : Gain  Gain=4
  I*R : Product  Inputs=**
  Ibty : Product  Inputs=*/
  R*Pbty : Product
  Sqrt : Sqrt  SaturateOnIntegerOverflow=on
  "Voc-I*R " : Sum  Inputs=+-
  Voc-sqrt : Sum  Inputs=+-
  Voc^2 : Product
  Voc^2 -4R*Pbty : Sum  Inputs=+-
  I [A] : Outport
  V [V] : Outport  Port=2
  wires:
  Output power [W]/1 -> R*Pbty/1
  Voc [V]/1 -> "Voc-I*R "/1, Voc-sqrt/1, Voc^2/2, Voc^2/1
  Rint [Ohm]/1 -> R*Pbty/2, 2*R/1, I*R/2
  R*Pbty/1 -> 4*R*Pbty/1
  Voc^2/1 -> Voc^2 -4R*Pbty/1
  4*R*Pbty/1 -> Voc^2 -4R*Pbty/2
  Voc^2 -4R*Pbty/1 -> Sqrt/1
  Sqrt/1 -> Voc-sqrt/2
  Voc-sqrt/1 -> Ibty/1
  2*R/1 -> Ibty/2
  Ibty/1 -> I [A]/1, I*R/1
  I*R/1 -> "Voc-I*R "/2
  "Voc-I*R "/1 -> V [V]/1

== system BugE_v0_40_MAS_loads_reg/Energy Storage (New Grid)/MB1/Energy Quantification ==
  V : Inport
  I : Inport  Port=2
  R : Inport  Port=3
  < 0 : Saturate  UpperLimit=0  LowerLimit=-inf
  > 0 : Saturate  UpperLimit=inf  LowerLimit=0  LinearizeAsGain=off
  Gain : Gain  Gain=-1
  Power : Product
  power loss : Product  Inputs=3
  tag scope: E_batt_loss1=global, E_batt_regen1=global, E_batt_useful1=global
  wires:
  V/1 -> Power/1
  I/1 -> Power/2, power loss/2, power loss/1
  Gain/1 -> [E_batt_regen1]
  Power/1 -> < 0/1, > 0/1
  < 0/1 -> Gain/1
  > 0/1 -> [E_batt_useful1]
  power loss/1 -> [E_batt_loss1]
  R/1 -> power loss/3

== system BugE_v0_40_MAS_loads_reg/Energy Storage (New Grid)/MB1/Pack Voc, R ==
  SOC_prev : Inport
  Req. power [W] : Inport  Port=2
  Temp [degC] : Inport  Port=3
  >=0 : simulink/Logic and Bit Operations/Compare To Zero  relop=>=  OutDataTypeStr=boolean
  Constant : Constant  Value=0.9  SampleTime=sample_time
  Constant1 : Constant  SampleTime=sample_time
  Product : Product  Inputs=3
  Product1 : Product  Inputs=/**/
  Product2 : Product  Inputs=/**/
  Product3 : Product
  R_charge [Ohm] : Lookup_n-D  BreakpointsForDimension1=ess_tmp  BreakpointsForDimension2=ess_soc  Table=ess_r_dis  InternalRulePriority=Speed  RndMeth=Simplest  InputSameDT=on
  R_discharge [Ohm] : Lookup_n-D  BreakpointsForDimension1=ess_tmp  BreakpointsForDimension2=ess_soc  Table=ess_r_dis  InternalRulePriority=Speed  RndMeth=Simplest  InputSameDT=on
  Switch : Switch  Criteria=u2 > Threshold
  Switch1 : Switch  Criteria=u2 > Threshold
  VOC [V] : Lookup_n-D  BreakpointsForDimension1=ess_tmp  BreakpointsForDimension2=ess_soc  Table=ess_voc  InternalRulePriority=Speed  RndMeth=Simplest  InputSameDT=on
  ess1_soh : Constant  Value=ess1_soh  SampleTime=sample_time
  ess_module _parallel : Constant  Value=ess_module_parallel  SampleTime=sample_time
  ess_module _series : Constant  Value=ess_module_series  SampleTime=sample_time
  Pack Voc [V] : Outport
  Pack R [Ohm] : Outport  Port=2
  wires:
  Switch/1 -> Pack R [Ohm]/1
  Req. power [W]/1 -> >=0/1
  R_discharge [Ohm]/1 -> Product1/2
  Product/1 -> Pack Voc [V]/1
  VOC [V]/1 -> Product/2
  ess_module _series/1 -> Product/3, Product2/2, Product1/3
  Temp [degC]/1 -> R_charge [Ohm]/1, R_discharge [Ohm]/1, VOC [V]/1
  SOC_prev/1 -> R_charge [Ohm]/2, R_discharge [Ohm]/2, VOC [V]/2
  Product3/1 -> Product2/1, Product1/1, Product/1
  >=0/1 -> Switch/2
  ess_module _parallel/1 -> Product1/4, Product2/4
  R_charge [Ohm]/1 -> Product2/3
  Product2/1 -> Switch/3
  Product1/1 -> Switch/1
  ess1_soh/1 -> Product3/2
  [MB1_lower_SOH] -> Switch1/2
  Constant/1 -> Switch1/1
  Constant1/1 -> Switch1/3
  Switch1/1 -> Product3/1

== system BugE_v0_40_MAS_loads_reg/Energy Storage (New Grid)/MB1 DCDC/Current limiter ==
  enable DCDC : Inport
  I batt side raw : Inport  Port=2
  I bus side raw : Inport  Port=3
  I max : Inport  Port=4
  " ==0 " : simulink/Logic and Bit Operations/Compare To Zero  relop===  OutDataTypeStr=boolean
  0 : Constant  Value=0  SampleTime=sample_time
  ==0 : simulink/Logic and Bit Operations/Compare To Zero  relop===  OutDataTypeStr=boolean
  Abs : Abs
  Abs1 : Abs
  Constant : Constant  SampleTime=sample_time
  Iin final : Product  Inputs=**
  Iin limited : Switch  Criteria=u2 > Threshold
  Iin over limit : RelationalOperator  Operator=>  OutDataTypeStr=boolean
  Iin raw avoid 0 div : Switch  Criteria=u2 > Threshold
  Imax : Product
  Iout final : Product  Inputs=**
  Iout limited : Switch  Criteria=u2 > Threshold
  Iout over limit : RelationalOperator  Operator=<  OutDataTypeStr=boolean
  Iout raw avoid 0 div : Switch  Criteria=u2 > Threshold
  Sign : Signum
  avoid 0 div2 : Switch  Criteria=u2 > Threshold
  avoid 0 div3 : Switch  Criteria=u2 > Threshold
  disable : Logic  Operator=NOT  AllPortsSameDT=off  OutDataTypeStr=boolean
  limit ratio : MinMax  Inputs=2
  limit ratio1 : Product  Inputs=*/
  limit ratio2 : Product  Inputs=*/
  or : Logic  Operator=OR  Inputs=3  AllPortsSameDT=off  OutDataTypeStr=boolean
  I batt side lim : Outport
  I bus side lim : Outport  Port=2
  wires:
  Iout raw avoid 0 div/1 -> Abs1/1, Iout final/2, limit ratio2/2, Iout limited/3
  Iin raw avoid 0 div/1 -> limit ratio1/2, Iin final/1, Iin limited/3, Sign/1, Abs/1
  Iin final/1 -> avoid 0 div2/3
  limit ratio2/1 -> limit ratio/2
  avoid 0 div3/1 -> I bus side lim/1
  Iin over limit/1 -> Iin limited/2
  Iout limited/1 -> limit ratio2/1
  Abs1/1 -> Iout over limit/2
  I max/1 -> Iin over limit/2, Imax/2, Iout over limit/1
  limit ratio/1 -> Iin final/2, Iout final/1
  Imax/1 -> Iin limited/1, Iout limited/1
  Abs/1 -> Iin over limit/1
  Sign/1 -> Imax/1
  limit ratio1/1 -> limit ratio/1
  Iin limited/1 -> limit ratio1/1
  Iout over limit/1 -> Iout limited/2
  I batt side raw/1 -> " ==0 "/1, Iin raw avoid 0 div/3
  enable DCDC/1 -> disable/1
  Constant/1 -> Iout raw avoid 0 div/1, Iin raw avoid 0 div/1
  I bus side raw/1 -> ==0/1, Iout raw avoid 0 div/3
  Iout final/1 -> avoid 0 div3/3
  0/1 -> avoid 0 div2/1, avoid 0 div3/1
  avoid 0 div2/1 -> I batt side lim/1
  or/1 -> avoid 0 div3/2, avoid 0 div2/2, Iin raw avoid 0 div/2, Iout raw avoid 0 div/2
  disable/1 -> or/3
  ==0/1 -> or/2
  " ==0 "/1 -> or/1

== system BugE_v0_40_MAS_loads_reg/Energy Storage (New Grid)/MB1 DCDC/Energy Quantification ==
  In1 : Inport
  In2 : Inport  Port=2
  In3 : Inport  Port=3
  In4 : Inport  Port=4
  Abs : Abs
  P lost : Sum  Inputs=-+
  Pin_DAB : Product
  Pout_DAB : Product
  tag scope: E_DAB1_loss=global
  wires:
  P lost/1 -> Abs/1
  In3/1 -> Pin_DAB/1
  Abs/1 -> [E_DAB1_loss]
  Pin_DAB/1 -> P lost/2
  Pout_DAB/1 -> P lost/1
  In4/1 -> Pin_DAB/2
  In2/1 -> Pout_DAB/2
  In1/1 -> Pout_DAB/1

== system BugE_v0_40_MAS_loads_reg/Energy Storage (New Grid)/MB1 DCDC/eff_maps ==
  "P into bus cmd " : Inport
  Vbus : Inport  Port=2
  Vbatt : Inport  Port=3
  1/V : Product  Inputs=*/
  >= eps : Saturate  UpperLimit=inf  LowerLimit=eps
  Demux : Demux  Outputs=2
  Divide : Product  Inputs=/*
  Gain : Gain  Gain=-1
  Interpolation: efficiency2 : Lookup_n-D  NumberOfTableDimensions=3  BreakpointsForDimension1=MC_Pouts  BreakpointsForDimension2=MC_Vins  BreakpointsForDimension3=MC_Vouts  Table=MC_eff2  InterpMethod=Cubic spline  InternalRulePriority=Speed  RndMeth=Simplest  InputSameDT=on
  Interpolation: efficiency1 : Lookup_n-D  NumberOfTableDimensions=3  BreakpointsForDimension1=MC_Pins  BreakpointsForDimension2=MC_Vins  BreakpointsForDimension3=MC_Vouts  Table=MC_eff1  InterpMethod=Cubic spline  InternalRulePriority=Speed  RndMeth=Simplest  InputSameDT=on
  Mux : Mux  Inputs=2
  Mux1 : Mux  Inputs=2
  Mux2 : Mux  Inputs=2
  P from batt : Switch
  Product : Product
  Saturation : Saturate  UpperLimit=MC_max_eff  LowerLimit=eps
  Saturation1 : Saturate  UpperLimit=MC_max_eff  LowerLimit=eps
  Switch1 : Switch
  I from batt & into bus : Outport
  wires:
  Vbus/1 -> Mux1/2, Mux/1
  Vbatt/1 -> Mux/2, Mux1/1
  Demux/2 -> Interpolation: efficiency1/3, Interpolation: efficiency2/3
  Mux/1 -> Switch1/3
  Switch1/1 -> Demux/1
  Gain/1 -> Interpolation: efficiency1/1
  Interpolation: efficiency2/1 -> Saturation/1
  Divide/1 -> P from batt/1
  Interpolation: efficiency1/1 -> Saturation1/1
  Product/1 -> P from batt/3
  P from batt/1 -> Mux2/1
  "P into bus cmd "/1 -> Gain/1, Interpolation: efficiency2/1, Switch1/2, Divide/2, Product/1, P from batt/2, Mux2/2
  Mux2/1 -> 1/V/1
  Mux1/1 -> >= eps/1, Switch1/1
  1/V/1 -> I from batt & into bus/1
  >= eps/1 -> 1/V/2
  Saturation/1 -> Divide/1
  Saturation1/1 -> Product/2
  Demux/1 -> Interpolation: efficiency2/2, Interpolation: efficiency1/2

== system BugE_v0_40_MAS_loads_reg/Energy Storage (New Grid)/MB1 DCDC/eff_maps1 ==
  I motor : Inport
  Vbatt cmd : Inport  Port=2
  Vbus : Inport  Port=3
  >= eps : Saturate  UpperLimit=inf  LowerLimit=eps
  Gain : Gain  Gain=-1
  I from bus : Product  Inputs=*//
  Interpolation: efficiency2 : Lookup_n-D  NumberOfTableDimensions=3  BreakpointsForDimension1=MC_Pouts  BreakpointsForDimension2=MC_Vins  BreakpointsForDimension3=MC_Vouts  Table=MC_eff2  InterpMethod=Cubic spline  InternalRulePriority=Speed  RndMeth=Simplest  InputSameDT=on
  Mux2 : Mux  Inputs=2
  P out to motor : Product
  Saturation : Saturate  UpperLimit=MC_max_eff  LowerLimit=eps
  I from batt & into bus : Outport
  wires:
  Interpolation: efficiency2/1 -> Saturation/1
  Mux2/1 -> Gain/1
  Gain/1 -> I from batt & into bus/1
  Vbus/1 -> >= eps/1
  Vbatt cmd/1 -> Interpolation: efficiency2/3, P out to motor/2
  I motor/1 -> Mux2/1, P out to motor/1
  P out to motor/1 -> Interpolation: efficiency2/1, I from bus/1
  I from bus/1 -> Mux2/2
  >= eps/1 -> I from bus/3, Interpolation: efficiency2/2
  Saturation/1 -> I from bus/2

== system BugE_v0_40_MAS_loads_reg/Energy Storage (New Grid)/MB2/Calculate SOC ==
  Temp [C] : Inport
  I [A] : Inport  Port=2
  1/3600 : Gain  Gain=1/3600
  Add : Sum  Inputs=-+
  Constant1 : Constant  SampleTime=sample_time
  Coulombic efficiency : Lookup_n-D  NumberOfTableDimensions=1  BreakpointsForDimension1=ess_tmp  Table=ess_coulombic_eff  InternalRulePriority=Speed  SaturateOnIntegerOverflow=on  InputSameDT=on
  Energy left [Ah] : Sum  Inputs=-+
  I adjusted : Product
  Max capacity [Ah] w/ SOH : Lookup_n-D  NumberOfTableDimensions=1  BreakpointsForDimension1=ess_tmp  Table=ess_max_ah_cap*ess2_soh  InternalRulePriority=Speed  SaturateOnIntegerOverflow=on  InputSameDT=on
  Multiply : Product
  Multiply1 : Product
  Resettable Integrator : Subsystem
  "SOC " : Product  Inputs=*/
  Saturation : Saturate  UpperLimit=1  LowerLimit=0
  Switch : Switch  Criteria=u2 > Threshold
  Switch1 : Switch  Criteria=u2 > Threshold
  ess_modules : Constant  Value=ess_module_series*ess_module_parallel  SampleTime=sample_time
  lockSOCs : Constant  Value=lockSOCs
  SOC : Outport
  wires:
  Resettable Integrator/1(Out1) -> Energy left [Ah]/1
  I [A]/1 -> Switch/2, Switch/1, I adjusted/1
  Switch/1 -> 1/3600/1
  Coulombic efficiency/1 -> I adjusted/2
  Energy left [Ah]/1 -> "SOC "/1
  I adjusted/1 -> Switch/3
  1/3600/1 -> Resettable Integrator/1(input)
  Temp [C]/1 -> Max capacity [Ah] w/ SOH/1, Coulombic efficiency/1
  Multiply1/1 -> "SOC "/2, Energy left [Ah]/2, Multiply/2
  "SOC "/1 -> Saturation/1
  Constant1/1 -> Add/2
  Multiply/1 -> Resettable Integrator/2(IC)
  Add/1 -> Multiply/1
  Switch1/1 -> SOC/1
  Max capacity [Ah] w/ SOH/1 -> Multiply1/1
  ess_modules/1 -> Multiply1/2
  [MB2_SOCinit] -> Switch1/1, Add/1
  Saturation/1 -> Switch1/3
  lockSOCs/1 -> Switch1/2

== system BugE_v0_40_MAS_loads_reg/Energy Storage (New Grid)/MB2/Compute current (nolimit) ==
  Voc [V] : Inport
  Rint [Ohm] : Inport  Port=2
  Output power [W] : Inport  Port=3
  2*R : Gain  Gain=2
  4*R*Pbty : Gain  Gain=4
  I*R : Product  Inputs=**
  Ibty : Product  Inputs=*/
  R*Pbty : Product
  Sqrt : Sqrt  SaturateOnIntegerOverflow=on
  "Voc-I*R " : Sum  Inputs=+-
  Voc-sqrt : Sum  Inputs=+-
  Voc^2 : Product
  Voc^2 -4R*Pbty : Sum  Inputs=+-
  I [A] : Outport
  V [V] : Outport  Port=2
  wires:
  Output power [W]/1 -> R*Pbty/1
  Voc [V]/1 -> "Voc-I*R "/1, Voc-sqrt/1, Voc^2/2, Voc^2/1
  Rint [Ohm]/1 -> R*Pbty/2, 2*R/1, I*R/2
  R*Pbty/1 -> 4*R*Pbty/1
  Voc^2/1 -> Voc^2 -4R*Pbty/1
  4*R*Pbty/1 -> Voc^2 -4R*Pbty/2
  Voc^2 -4R*Pbty/1 -> Sqrt/1
  Sqrt/1 -> Voc-sqrt/2
  Voc-sqrt/1 -> Ibty/1
  2*R/1 -> Ibty/2
  Ibty/1 -> I [A]/1, I*R/1
  I*R/1 -> "Voc-I*R "/2
  "Voc-I*R "/1 -> V [V]/1

== system BugE_v0_40_MAS_loads_reg/Energy Storage (New Grid)/MB2/Energy Quantification ==
  In2 : Inport
  In3 : Inport  Port=2
  In1 : Inport  Port=3
  < 0 : Saturate  UpperLimit=0  LowerLimit=-inf
  > 0 : Saturate  UpperLimit=inf  LowerLimit=0  LinearizeAsGain=off
  Gain : Gain  Gain=-1
  Power : Product
  power loss : Product  Inputs=3
  tag scope: E_batt_loss2=global, E_batt_regen2=global, E_batt_useful2=global
  wires:
  In2/1 -> Power/1
  In3/1 -> Power/2, power loss/2, power loss/1
  Gain/1 -> [E_batt_regen2]
  Power/1 -> < 0/1, > 0/1
  < 0/1 -> Gain/1
  > 0/1 -> [E_batt_useful2]
  power loss/1 -> [E_batt_loss2]
  In1/1 -> power loss/3

== system BugE_v0_40_MAS_loads_reg/Energy Storage (New Grid)/MB2/Pack Voc, R ==
  SOC_prev : Inport
  Req. power [W] : Inport  Port=2
  Temp [degC] : Inport  Port=3
  >=0 : simulink/Logic and Bit Operations/Compare To Zero  relop=>=  OutDataTypeStr=boolean
  Product : Product  Inputs=3
  Product1 : Product  Inputs=/**/
  Product2 : Product  Inputs=/**/
  R_charge [Ohm] : Lookup_n-D  BreakpointsForDimension1=ess_tmp  BreakpointsForDimension2=ess_soc  Table=ess_r_dis  InternalRulePriority=Speed  RndMeth=Simplest  InputSameDT=on
  R_discharge [Ohm] : Lookup_n-D  BreakpointsForDimension1=ess_tmp  BreakpointsForDimension2=ess_soc  Table=ess_r_dis  InternalRulePriority=Speed  RndMeth=Simplest  InputSameDT=on
  Switch : Switch  Criteria=u2 > Threshold
  VOC [V] : Lookup_n-D  BreakpointsForDimension1=ess_tmp  BreakpointsForDimension2=ess_soc  Table=ess_voc  InternalRulePriority=Speed  RndMeth=Simplest  InputSameDT=on
  ess2_soh : Constant  Value=ess2_soh  SampleTime=sample_time
  ess_module _parallel : Constant  Value=ess_module_parallel  SampleTime=sample_time
  ess_module _series : Constant  Value=ess_module_series  SampleTime=sample_time
  Pack Voc [V] : Outport
  Pack R [Ohm] : Outport  Port=2
  wires:
  Switch/1 -> Pack R [Ohm]/1
  Req. power [W]/1 -> >=0/1
  R_discharge [Ohm]/1 -> Product1/2
  Product/1 -> Pack Voc [V]/1
  VOC [V]/1 -> Product/2
  ess_module _series/1 -> Product/3, Product2/2, Product1/3
  Temp [degC]/1 -> R_charge [Ohm]/1, R_discharge [Ohm]/1, VOC [V]/1
  SOC_prev/1 -> R_charge [Ohm]/2, R_discharge [Ohm]/2, VOC [V]/2
  ess2_soh/1 -> Product2/1, Product1/1, Product/1
  >=0/1 -> Switch/2
  ess_module _parallel/1 -> Product1/4, Product2/4
  R_charge [Ohm]/1 -> Product2/3
  Product2/1 -> Switch/3
  Product1/1 -> Switch/1

== system BugE_v0_40_MAS_loads_reg/Energy Storage (New Grid)/MB2 DCDC/Current limiter ==
  enable DCDC : Inport
  I batt side raw : Inport  Port=2
  I bus side raw : Inport  Port=3
  I max : Inport  Port=4
  " ==0 " : simulink/Logic and Bit Operations/Compare To Zero  relop===  OutDataTypeStr=boolean
  0 : Constant  Value=0  SampleTime=sample_time
  ==0 : simulink/Logic and Bit Operations/Compare To Zero  relop===  OutDataTypeStr=boolean
  Abs : Abs
  Abs1 : Abs
  Constant : Constant  SampleTime=sample_time
  Iin final : Product  Inputs=**
  Iin limited : Switch  Criteria=u2 > Threshold
  Iin over limit : RelationalOperator  Operator=>  OutDataTypeStr=boolean
  Iin raw avoid 0 div : Switch  Criteria=u2 > Threshold
  Imax : Product
  Iout final : Product  Inputs=**
  Iout limited : Switch  Criteria=u2 > Threshold
  Iout over limit : RelationalOperator  Operator=<  OutDataTypeStr=boolean
  Iout raw avoid 0 div : Switch  Criteria=u2 > Threshold
  Sign : Signum
  avoid 0 div2 : Switch  Criteria=u2 > Threshold
  avoid 0 div3 : Switch  Criteria=u2 > Threshold
  disable : Logic  Operator=NOT  AllPortsSameDT=off  OutDataTypeStr=boolean
  limit ratio : MinMax  Inputs=2
  limit ratio1 : Product  Inputs=*/
  limit ratio2 : Product  Inputs=*/
  or : Logic  Operator=OR  Inputs=3  AllPortsSameDT=off  OutDataTypeStr=boolean
  I batt side lim : Outport
  I bus side lim : Outport  Port=2
  wires:
  Iout raw avoid 0 div/1 -> Abs1/1, Iout final/2, limit ratio2/2, Iout limited/3
  Iin raw avoid 0 div/1 -> limit ratio1/2, Iin final/1, Iin limited/3, Sign/1, Abs/1
  Iin final/1 -> avoid 0 div2/3
  limit ratio2/1 -> limit ratio/2
  avoid 0 div3/1 -> I bus side lim/1
  Iin over limit/1 -> Iin limited/2
  Iout limited/1 -> limit ratio2/1
  Abs1/1 -> Iout over limit/2
  I max/1 -> Iin over limit/2, Imax/2, Iout over limit/1
  limit ratio/1 -> Iin final/2, Iout final/1
  Imax/1 -> Iin limited/1, Iout limited/1
  Abs/1 -> Iin over limit/1
  Sign/1 -> Imax/1
  limit ratio1/1 -> limit ratio/1
  Iin limited/1 -> limit ratio1/1
  Iout over limit/1 -> Iout limited/2
  I batt side raw/1 -> " ==0 "/1, Iin raw avoid 0 div/3
  enable DCDC/1 -> disable/1
  Constant/1 -> Iout raw avoid 0 div/1, Iin raw avoid 0 div/1
  I bus side raw/1 -> ==0/1, Iout raw avoid 0 div/3
  Iout final/1 -> avoid 0 div3/3
  0/1 -> avoid 0 div2/1, avoid 0 div3/1
  avoid 0 div2/1 -> I batt side lim/1
  or/1 -> avoid 0 div3/2, avoid 0 div2/2, Iin raw avoid 0 div/2, Iout raw avoid 0 div/2
  disable/1 -> or/3
  ==0/1 -> or/2
  " ==0 "/1 -> or/1

== system BugE_v0_40_MAS_loads_reg/Energy Storage (New Grid)/MB2 DCDC/Energy Quantification ==
  In1 : Inport
  In2 : Inport  Port=2
  In3 : Inport  Port=3
  In4 : Inport  Port=4
  Abs : Abs
  P lost : Sum  Inputs=-+
  Pin_DAB : Product
  Pout_DAB : Product
  tag scope: E_DAB2_loss=global
  wires:
  P lost/1 -> Abs/1
  In3/1 -> Pin_DAB/1
  Abs/1 -> [E_DAB2_loss]
  Pin_DAB/1 -> P lost/2
  Pout_DAB/1 -> P lost/1
  In4/1 -> Pin_DAB/2
  In2/1 -> Pout_DAB/2
  In1/1 -> Pout_DAB/1
